simulink model "MotorModel"  (R2020b)
settings: Solver=VariableStepAuto  StartTime=0.0  StopTime=10.0  RelTol=1e-3  EnableMultiTasking=on
undefined symbols (not defined in the file or in its folder): Initial, Motor, Uav
settings Model: Creator=jban039  LastModifiedBy=jeremie
settings DataIOCC: LimitDataPoints=on
settings OptimizationCC: LifeSpan=inf
settings DebuggingCC: AllowSymbolicDim=off  SFUnexpectedBacktrackingDiag=warning  SFNoUnconditionalDefaultTransitionDiag=warning  SFExecutionAtInitializationDiag=none  ArithmeticOperatorsInVariantConditions=warning
settings ModelReferenceCC: PropagateSignalLabelsOutOfModel=off
settings SFSimCC: SimUseLocalCustomCode=off  CustomCodeUndefinedFunction=UseInterfaceOnly
settings RTWCC: RTWUseLocalCustomCode=off
settings CodeAppCC: StateflowObjectComments=on
settings GRTTargetCC: TargetLangStandard=C89/C90 (ANSI)
settings ConfigComp: CovMetricSettings=dw  CovSaveCumulativeToWorkspaceVar=on  CovSaveSingleToWorkspaceVar=on  CovExternalEMLEnable=off

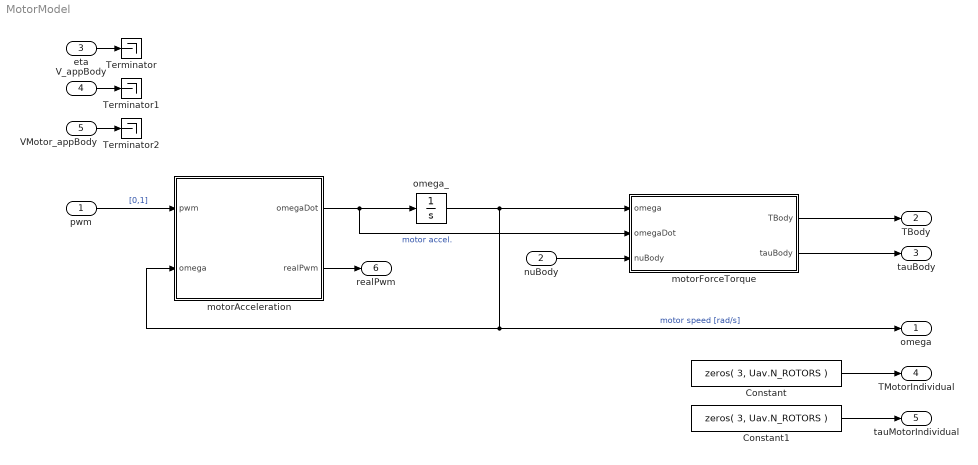
== system MotorModel ==
  pwm : Inport  PortDimensions=Uav.N_ROTORS
  nuBody : Inport  Port=2
  eta : Inport  Port=3  Unit=rad  PortDimensions=3
  V_appBody : Inport  Port=4  Unit=m/s  PortDimensions=3
  VMotor_appBody : Inport  Port=5  Unit=m/s  PortDimensions=[3,Uav.N_ROTORS]
  Constant : Constant  Value=zeros( 3, Uav.N_ROTORS )
  Constant1 : Constant  Value=zeros( 3, Uav.N_ROTORS )
  Terminator : Terminator
  Terminator1 : Terminator
  Terminator2 : Terminator
  motorAcceleration : MATLAB Function  TreatAsAtomicUnit=on
  motorForceTorque : MATLAB Function  TreatAsAtomicUnit=on
  omega_ : Integrator  InitialCondition=Initial.OMEGA  LimitOutput=on  LowerSaturationLimit=zeros(size(Initial.OMEGA))  ContinuousStateAttributes='omega'
  omega : Outport  Unit=rad/s  VectorParamsAs1DForOutWhenUnconnected=off
  TBody : Outport  Port=2  Unit=N  VectorParamsAs1DForOutWhenUnconnected=off
  tauBody : Outport  Port=3  Unit=N*m  VectorParamsAs1DForOutWhenUnconnected=off
  TMotorIndividual : Outport  Port=4  Unit=N  VectorParamsAs1DForOutWhenUnconnected=off
  tauMotorIndividual : Outport  Port=5  Unit=N*m  VectorParamsAs1DForOutWhenUnconnected=off
  realPwm : Outport  Port=6  VectorParamsAs1DForOutWhenUnconnected=off
  wires:
  motorAcceleration/1(omegaDot) -> motorForceTorque/2(omegaDot), omega_/1  "motor accel."
  motorForceTorque/2(tauBody) -> tauBody/1
  motorForceTorque/1(TBody) -> TBody/1
  omega_/1 -> motorForceTorque/1(omega), motorAcceleration/2(omega), omega/1  "motor speed [rad/s]"
  pwm/1 -> motorAcceleration/1(pwm)  "[0,1]"
  nuBody/1 -> motorForceTorque/3(nuBody)
  eta/1 -> Terminator/1
  V_appBody/1 -> Terminator1/1
  Constant/1 -> TMotorIndividual/1
  VMotor_appBody/1 -> Terminator2/1
  motorAcceleration/2(realPwm) -> realPwm/1
  Constant1/1 -> tauMotorIndividual/1

== matlab function MotorModel/motorForceTorque ==
  data: omega input; TBody output size=3; omegaDot input; nuBody input size=3; Motor parameter; Uav parameter; tauBody output size=3
function [TBody, tauBody] = motorForceTorque(...
    omega, omegaDot, nuBody, Motor, Uav)
%#codegen

% Make assertions to avoid code generation errors
assert(Uav.N_ROTORS < 16);

%% Thrust and differential torque

% Concatenated motor force/torque vectors in respective motor frame
% eg. TMotor = [TMotor1, TMotor2, ..., TMotorN]
% where: - N is the number of rotors
%        - TMotorx (x ∈ [1,2,...,N]) is the thrust generated by motor x in
%          its own frame of reference
TMotorIndividual = [ 0*omega'; 0*omega'; % Avoid using zeros(1,Uav.N_ROTORS), which causes issues
           -Motor.K .* (omega'.^2) ];
tauMotorIndividual = [ 0*omega'; 0*omega';
             -Uav.ROTOR_DIRECTION .* ...
                 ( Motor.B.*(omega'.^2) + Motor.I_R_ZZ.*omegaDot' ) ];

% Initialise matrices to store motor force/torque vectors in body frame
TBodyIndividual   = zeros(3, Uav.N_ROTORS);
tauBodyIndividual = zeros(3, Uav.N_ROTORS);

% Calculate forces and moments from each motor in the body frame
for i = 1:Uav.N_ROTORS
    l = Uav.L(i);
    beta = Uav.BETA(i);
    
    % Matrix to compute torque applied by rotor thrust
 	L = [ 0,            0,            l*sin(beta);
          0,            0,           -l*cos(beta);
         -l*sin(beta),  l*cos(beta),  0 ];

	% Motor force/torque vectors in body frame
	TBodyIndividual(:,i) = Uav.R_MOTOR_TO_BODY(:,:,i) * ...
        TMotorIndividual(:,i);
	tauBodyIndividual(:,i) = Uav.R_MOTOR_TO_BODY(:,:,i) * ...
        tauMotorIndividual(:,i) + L * TBodyIndividual(:,i);
end

%% Gyroscopic moments

% Concatenated gyroscopic moments for each rotor
M_GBodyIndividual = [0*omega'; 0*omega'; 0*omega'];
H_MMotorSeparate = [0*omega'; 0*omega'; 0*omega'];

% Concatenated motor speeds in their respective frames
omegaMotor = [ 0*omega'; 0*omega';
               Uav.ROTOR_DIRECTION .* omega' ];
           
for i = 1:Uav.N_ROTORS
    % Angular momentum in motor frame
    H_MMotorSeparate(:,i) = Motor.I_R(:,:,i) * omegaMotor(:,i);

    % Gyroscopic moment vectors in body frame
	M_GBodyIndividual(:,i) = cross( nuBody, ...
        Uav.R_MOTOR_TO_BODY(:,:,i) * H_MMotorSeparate(:,i) );
end

M_GBody = sum(M_GBodyIndividual, 2);

%% Total torque and moment

% Total force/torque in body frame
TBody = sum(TBodyIndividual, 2);
tauBody = sum(tauBodyIndividual, 2) - M_GBody;

end

== matlab function MotorModel/motorAcceleration ==
  data: pwm input; omegaDot output double; omega input; realPwm output
function [omegaDot, realPwm]  = motorRotDynamics( pwm, omega )
%#codegen

realPwm = (1000 * pwm + 1000);

rotorTimeConst = 7.006512e-02;
omegaRef = 0.84 * ( 7.969173e-1.*realPwm - 6.528579e2 );

omegaDot = (omegaRef - omega) / rotorTimeConst;
end
